simulink model "sim_integr"  (R2022b)
settings: Solver=VariableStepAuto  StartTime=0.0  StopTime=10  RelTol=1e-3
settings Model: Creator=isaac  LastModifiedBy=isaac
settings DebuggingCC: UnconnectedInputMsg=warning  UnconnectedOutputMsg=warning  UnconnectedLineMsg=warning
settings ModelReferenceCC: EnableRefExpFcnMdlSchedulingChecks=on
settings RTWCC: DLArmComputeVersion=19.05

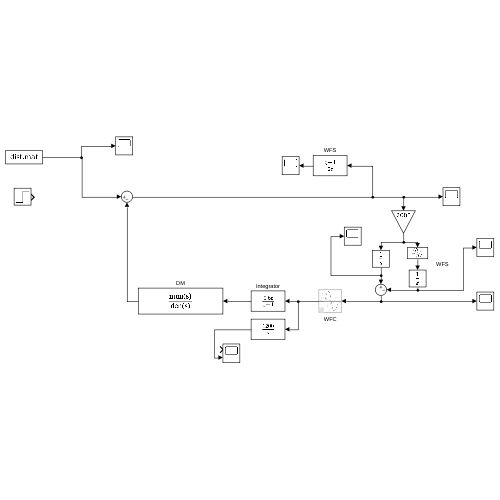
[thumbnail: Simulink's stored preview of the top-level diagram]
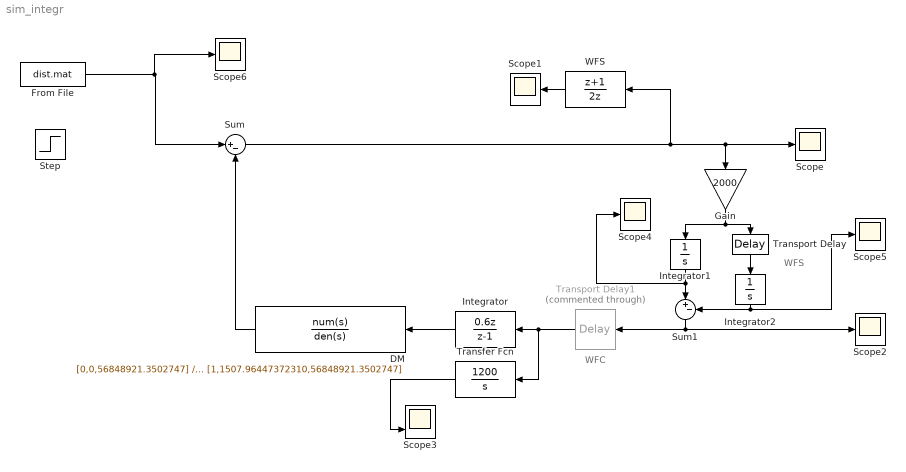
== system sim_integr ==
  note: WFC
  note: WFS
  DM : TransferFcn  Tag=DM  Numerator=[0,0,56848921.3502747]  Denominator=[1,1507.96447372310,56848921.3502747]
  From File : FromFile  FileName=dist.mat  SampleTime=0.0005  ExtrapolationBeforeFirstDataPoint=Ground value  ExtrapolationAfterLastDataPoint=Ground value
  Gain : Gain  Gain=2000
  Integrator : DiscreteTransferFcn  Numerator=[0.6 0]  Denominator=[1 -1]  SampleTime=0.0005
  Integrator1 : Integrator
  Integrator2 : Integrator
  Scope{,1..2,4..6} (6 alike) : Scope
  Scope3 : Scope  NumInputPorts=2
  Step : Step  Before=1  SampleTime=0
  Sum : Sum  Inputs=|+-
  Sum1 : Sum  Inputs=|+-
  Transfer Fcn : TransferFcn  Numerator=[1200]  Denominator=[1 0]
  Transport Delay : TransportDelay  DelayTime=0.0005
  Transport Delay1 : TransportDelay  Commented=through  DelayTime=0.00065
  WFS : DiscreteTransferFcn  Numerator=[1 1]  Denominator=[2 0]
  wires:
  Sum/1 -> Scope/1, Gain/1, WFS/1
  WFS/1 -> Scope1/1
  Transport Delay/1 -> Integrator2/1
  Integrator1/1 -> Scope4/1, Sum1/1
  Integrator2/1 -> Scope5/1, Sum1/2
  Gain/1 -> Integrator1/1, Transport Delay/1
  DM/1 -> Sum/2
  Transport Delay1/1 -> Transfer Fcn/1, Integrator/1
  Transfer Fcn/1 -> Scope3/2
  Sum1/1 -> Transport Delay1/1, Scope2/1
  From File/1 -> Scope6/1, Sum/1
  Integrator/1 -> DM/1
